simulink model "Helicopter_sol"  (R2023b)
settings: Solver=ode3  StartTime=0.0  StopTime=20  FixedStep=0.01  RelTol=1e-3
undefined symbols (not defined in the file): A, B, K, N_bar
libraries: simulink_extras x3
settings Model: Creator=jerome  LastModifiedBy=jerome
settings ModelReferenceCC: EnableRefExpFcnMdlSchedulingChecks=on

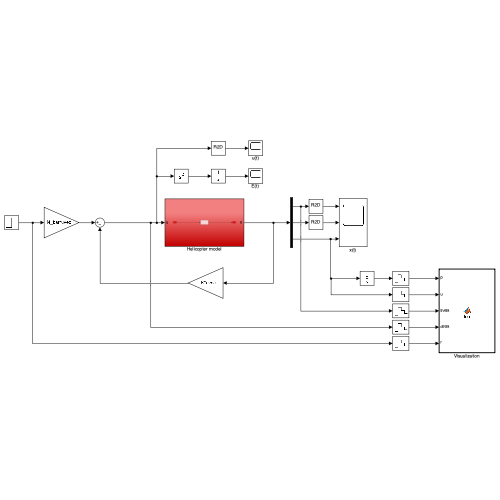
[thumbnail: Simulink's stored preview of the top-level diagram]
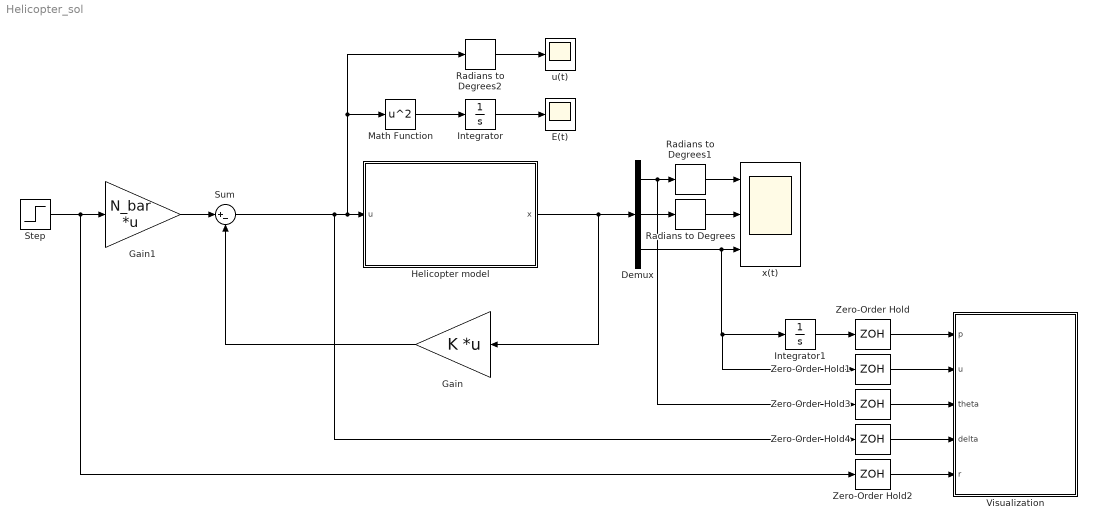
== system Helicopter_sol ==
  Demux : Demux  Outputs=3
  E(t) : Scope
  Gain : Gain  Gain=K  Multiplication=Matrix(K*u) (u vector)
  Gain1 : Gain  Gain=N_bar  Multiplication=Matrix(K*u) (u vector)
  Helicopter model : Subsystem
  Integrator : Integrator
  Integrator1 : Integrator
  Math Function : Math  Operator=square
  Radians to Degrees : simulink_extras/Transformations/Radians to Degrees
  Radians to Degrees1 : simulink_extras/Transformations/Radians to Degrees
  Radians to Degrees2 : simulink_extras/Transformations/Radians to Degrees
  Step : Step  Time=0  After=10  SampleTime=0
  Sum : Sum  Inputs=|+-
  Visualization : MATLAB Function  TreatAsAtomicUnit=on
  Zero-Order Hold{,1..4} (5 alike) : ZeroOrderHold  SampleTime=0.1
  u(t) : Scope
  x(t) : Scope  NumInputPorts=3
  wires:
  Helicopter model/1(x) -> Gain/1, Demux/1
  Gain/1 -> Sum/2
  Gain1/1 -> Sum/1
  Integrator/1 -> E(t)/1
  Math Function/1 -> Integrator/1
  Demux/2 -> Radians to Degrees/1
  Radians to Degrees/1 -> x(t)/2
  Radians to Degrees1/1 -> x(t)/1
  Radians to Degrees2/1 -> u(t)/1
  Demux/3 -> Zero-Order Hold1/1, Integrator1/1, x(t)/3
  Integrator1/1 -> Zero-Order Hold/1
  Zero-Order Hold3/1 -> Visualization/3(theta)
  Zero-Order Hold4/1 -> Visualization/4(delta)
  Step/1 -> Zero-Order Hold2/1, Gain1/1
  Zero-Order Hold1/1 -> Visualization/2(u)
  Zero-Order Hold/1 -> Visualization/1(p)
  Demux/1 -> Zero-Order Hold3/1, Radians to Degrees1/1
  Zero-Order Hold2/1 -> Visualization/5(r)
  Sum/1 -> Zero-Order Hold4/1, Helicopter model/1(u), Math Function/1, Radians to Degrees2/1

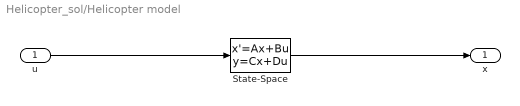
== system Helicopter_sol/Helicopter model ==
  u : Inport
  State-Space : StateSpace  A=A  B=B  C=eye(3)  D=zeros(3,1)  InitialCondition=[0;0;0]
  x : Outport
  wires:
  u/1 -> State-Space/1
  State-Space/1 -> x/1

== matlab function Helicopter_sol/Visualization ==
  data: p input; u input; theta input; delta input; r input
function fcn(p,u,theta,delta,r)


% body
    Xbody = [ 1 ; -3 ; -3 ; -6 ; -6.5 ; -7.5 ; -7 ; -7 ; -6.7 ; -6.3 ; -6 ; -3 ; -2 ; 2 ;3 ;4 ; 4 ; 1.2 ];
    Ybody = [ 1 ; 1 ; 0.5 ; 0.8 ; 2 ; 2; 0.8 ; 0 ; -0.4 ; -0.4 ; 0 ; -0.5 ; -1 ; -1 ; -0.8 ; -0.4 ; 0 ; 0]; 

% canopy
    Xcanopy = [ 1.2 ; 3.9 ; 2.9 ; 1 ];
    Ycanopy = [ 0 ; 0 ; 0.8 ; 0.9 ];
    
% rotor
    Xrotor = [ 0.6 ; 0.6; 0.2 ; 0.2 ; -0.2 ; -0.2 ; -0.6 ; -0.6 ];
    Yrotor = [ 1 ; 2 ; 2 ; 3 ; 3 ; 2; 2; 1 ];

% propeller
    Xprop = [ -5 ; 5 ];
    Yprop = [ 0 ; 0];
    

% calculate graphical position of helicopter
      [PosXbody,PosYbody] = rot(Xbody,Ybody,-theta);
      PosXbody = PosXbody + p;
      PosYbody = PosYbody + 10;

      [PosXcanopy,PosYcanopy] = rot(Xcanopy,Ycanopy,-theta);
      PosXcanopy = PosXcanopy + p;
      PosYcanopy = PosYcanopy + 10;

      [PosXrotor,PosYrotor] = rot(Xrotor,Yrotor,-theta);
      PosXrotor = PosXrotor + p;
      PosYrotor = PosYrotor + 10;

      [PosXprop,PosYprop] = rot(Xprop,Yprop,-delta);
      PosXprop = PosXprop ;
      PosYprop = PosYprop + 3;
      [PosXprop,PosYprop] = rot(PosXprop,PosYprop,-theta);
      PosXprop = PosXprop + p;
      PosYprop = PosYprop + 10;

      if r == 0
         r_normed = 0;
      else
         r_normed = r/abs(r);
      end


% to be able to use 'fill' even though the function is not supported for code generation
% see https://se.mathworks.com/help/simulink/slref/coder.extrinsic.html
coder.extrinsic('fill'); 

% draw the body of the helicopter with the proper position and orientation
fill(PosXbody,PosYbody,'g'); % put my green instead

hold on
% draw the rest of the helicopter
fill(PosXcanopy,PosYcanopy,'b');
fill(PosXrotor,PosYrotor,'k');
line(PosXprop,PosYprop,'Color','r','LineWidth',4);
quiver(p,2,5*r_normed,0, 'AutoScale','off','LineWidth',2,'Color','b'); % represent normalized reference
quiver(p,4,5*u/max(abs(r),1e-6),0, 'AutoScale','off','LineWidth',2,'Color','r'); % represent ratio between u and r

hold off

if p <= 4
    axis([-10 10 0 20]);
else
    axis([p-14 p+6 0 20]);
end

%axis([-10 10 0 20]);
title('Helicopter cruise control', 'FontSize',20);
axis square;
grid on;

drawnow;



% function "rot" that rotates a graphical object
function [PosX,PosY] = rot(X,Y,angle)

dim = size(X,1);
PosX = zeros(dim,1);
PosY = zeros(dim,1);

Mrot = [ cos(angle) -sin(angle)  ;
         sin(angle)  cos(angle) ]; 

for i=1:dim
    Pos_i = Mrot * [ X(i,1) ; Y(i,1) ];
    PosX(i,1) = Pos_i(1,1);
    PosY(i,1) = Pos_i(2,1);
end
